simulink model "Quadcopter_Sim"  (R2020b)
settings: Solver=VariableStepAuto  StartTime=0.0  StopTime=32  RelTol=1e-3
values from neighbouring files (symbols this model uses):
  b = 1.14*10^-7    (= 1.14e-07)    [Quadcopter_Code.m]
  g = 9.81    [Quadcopter_Code.m]
  Ix = 4.856 * 10^-3    (= 0.004856)    [Quadcopter_Code.m]
  Iy = 4.856 * 10^-3    (= 0.004856)    [Quadcopter_Code.m]
  Iz = 8.801*10^-3    (= 0.008801)    [Quadcopter_Code.m]
  k = 2.98*10^-6    (= 2.98e-06)    [Quadcopter_Code.m]
  l = 0.225    [Quadcopter_Code.m]
  m = 0.468    [Quadcopter_Code.m]
libraries: pid_lib x2
settings Model: Creator=ethan  LastModifiedBy=ethan
settings OptimizationCC: BlockReduction=off  DefaultParameterBehavior=Inlined  BufferReuse=off

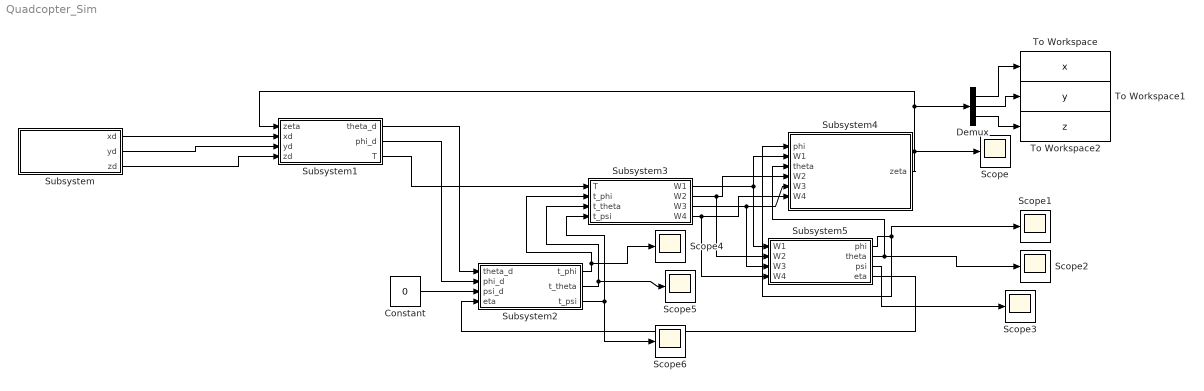
== system Quadcopter_Sim ==
  Constant : Constant  Value=0
  Demux : Demux  Outputs=3
  Scope{,1..6} (7 alike) : Scope
  Subsystem : Subsystem
  Subsystem1 : Subsystem
  Subsystem2 : Subsystem
  Subsystem3 : Subsystem
  Subsystem4 : Subsystem
  Subsystem5 : Subsystem
  To Workspace : ToWorkspace  VariableName=x  SaveFormat=Timeseries  SampleTime=-1
  To Workspace1 : ToWorkspace  VariableName=y  SaveFormat=Timeseries  SampleTime=-1
  To Workspace2 : ToWorkspace  VariableName=z  SaveFormat=Timeseries  SampleTime=-1
  wires:
  Subsystem/1(xd) -> Subsystem1/2(xd)
  Subsystem/2(yd) -> Subsystem1/3(yd)
  Subsystem/3(zd) -> Subsystem1/4(zd)
  Constant/1 -> Subsystem2/3(psi_d)
  Subsystem1/2(phi_d) -> Subsystem2/2(phi_d)
  Subsystem1/1(theta_d) -> Subsystem2/1(theta_d)
  Subsystem1/3(T) -> Subsystem3/1(T)
  Subsystem3/1(W1) -> Subsystem5/1(W1), Subsystem4/2(W1)
  Subsystem5/1(phi) -> Scope1/1, Subsystem4/1(phi)
  Subsystem4/1(zeta) -> Subsystem1/1(zeta), Demux/1, Scope/1
  Subsystem5/2(theta) -> Scope2/1, Subsystem4/3(theta)
  Subsystem5/3(psi) -> Scope3/1
  Subsystem5/4(eta) -> Subsystem2/4(eta)
  Subsystem2/1(t_phi) -> Scope4/1, Subsystem3/2(t_phi)
  Subsystem2/2(t_theta) -> Scope5/1, Subsystem3/3(t_theta)
  Subsystem2/3(t_psi) -> Subsystem3/4(t_psi), Scope6/1
  Subsystem3/2(W2) -> Subsystem5/2(W2), Subsystem4/4(W2)
  Subsystem3/3(W3) -> Subsystem4/5(W3), Subsystem5/3(W3)
  Subsystem3/4(W4) -> Subsystem5/4(W4), Subsystem4/6(W4)
  Demux/1 -> To Workspace/1
  Demux/2 -> To Workspace1/1
  Demux/3 -> To Workspace2/1

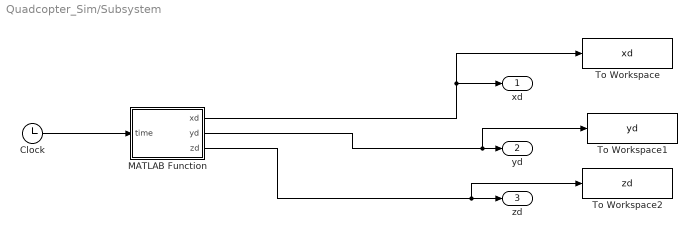
== system Quadcopter_Sim/Subsystem ==
  Clock : Clock
  MATLAB Function : MATLAB Function  TreatAsAtomicUnit=on
  To Workspace : ToWorkspace  VariableName=xd  SaveFormat=Timeseries  SampleTime=-1
  To Workspace1 : ToWorkspace  VariableName=yd  SaveFormat=Timeseries  SampleTime=-1
  To Workspace2 : ToWorkspace  VariableName=zd  SaveFormat=Timeseries  SampleTime=-1
  xd : Outport
  yd : Outport  Port=2
  zd : Outport  Port=3
  wires:
  MATLAB Function/1(xd) -> To Workspace/1, xd/1
  MATLAB Function/2(yd) -> To Workspace1/1, yd/1
  MATLAB Function/3(zd) -> To Workspace2/1, zd/1
  Clock/1 -> MATLAB Function/1(time)

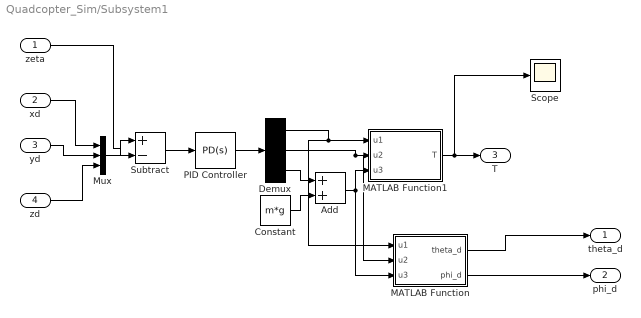
== system Quadcopter_Sim/Subsystem1 ==
  zeta : Inport
  xd : Inport  Port=2
  yd : Inport  Port=3
  zd : Inport  Port=4
  Add : Sum
  Constant : Constant  Value=m*g
  Demux : Demux  Outputs=3
  MATLAB Function : MATLAB Function  TreatAsAtomicUnit=on
  MATLAB Function1 : MATLAB Function  TreatAsAtomicUnit=on
  Mux : Mux  Inputs=3
  PID Controller : pid_lib/PID Controller  Controller=PD  Form=Parallel  TimeDomain=Continuous-time  UseExternalTs=off  SampleTime=-1  IntegratorMethod=Forward Euler  FilterMethod=Forward Euler  ControllerParametersSource=internal  P=4  I=0  D=2  UseFilter=on  N=100  TunerSelectOption=Transfer Function Based (PID Tuner App)  InitialConditionSource=internal  InitialConditionForIntegrator=0  InitialConditionForFilter=0  DifferentiatorICPrevScaledInput=0  ExternalReset=none  TrackingMode=off  Kt=1  LimitOutput=off  SatLimitsSource=internal  UpperSaturationLimit=inf  LowerSaturationLimit=-inf  LinearizeAsGain=on  AntiWindupMode=none  Kb=1  POutMin=[]  POutMax=[]  IOutMin=[]  IOutMax=[]  DOutMin=[]  DOutMax=[]  NOutMin=[]  NOutMax=[]  SumOutMin=[]  SumOutMax=[]  SaturationOutMin=[]  SaturationOutMax=[]  PParamMin=[]  PParamMax=[]  IParamMin=[]  IParamMax=[]  DParamMin=[]  DParamMax=[]  NParamMin=[]  NParamMax=[]  KbParamMin=[]  KbParamMax=[]  KtParamMin=[]  KtParamMax=[]  KbOutMin=[]  KbOutMax=[]  KtOutMin=[]  KtOutMax=[]  IntegratorOutMin=[]  IntegratorOutMax=[]  FilterOutMin=[]  FilterOutMax=[]  SumI1OutMin=[]  SumI1OutMax=[]  SumI2OutMin=[]  SumI2OutMax=[]  SumI3OutMin=[]  SumI3OutMax=[]  SumI4OutMin=[]  SumI4OutMax=[]  SumDOutMin=[]  SumDOutMax=[]  DifferentiatorOutMin=[]  DifferentiatorOutMax=[]  FilterDiffOutCoefMin=[]  FilterDiffOutCoefMax=[]  ReciprocalOutMin=[]  ReciprocalOutMax=[]  SumDenOutMin=[]  SumDenOutMax=[]  SumNumOutMin=[]  SumNumOutMax=[]  DivideOutMin=[]  DivideOutMax=[]  UdiffTsProdOutMin=[]  UdiffTsProdOutMax=[]  NTsProdOutMin=[]  NTsProdOutMax=[]  UintegralTsProdOutMin=[]  UintegralTsProdOutMax=[]  UngainTsProdOutMin=[]  UngainTsProdOutMax=[]  IntegratorContinuousStateAttributes=''  IntegratorStateMustResolveToSignalObject=off  IntegratorRTWStateStorageClass=Auto  FilterContinuousStateAttributes=''  FilterStateMustResolveToSignalObject=off  FilterRTWStateStorageClass=Auto  ParallelPVariant=InternalParameters  IdealPVariant=Disabled  IVariant=Disabled  DVariant=InternalParameters  IntegratorVariant=Disabled  SatVariant=Disabled  AWVariant=Disabled  PCopyVariant=Disabled  TRVariant=Disabled  FdbkBlocksVariant=Forward  IdealPFdbkVariant=Disabled  SatFdbkVariant=Disabled  DerivativeFilterVariant=ContFilter  NVariant=InternalParameters  NCopyVariant=Disabled  FilterICVariant=InternalICsFilter  IntegratorICVariant=Disabled  ExternalResetVariant=Disabled  TRSumVariant=Passthrough  SumFdbkVariant=Disabled  SumVariant=Sum_PD  TsampFilterVariant=InternalTs  TsampNgainVariant=Passthrough  TsampIntegralVariant=Disabled_SignalSpec  ExternalSaturationOutDataTypeStr=Inherit: Same as second input
  Scope : Scope
  Subtract : Sum  Inputs=+-
  theta_d : Outport
  phi_d : Outport  Port=2
  T : Outport  Port=3
  wires:
  xd/1 -> Mux/1
  yd/1 -> Mux/2
  zd/1 -> Mux/3
  zeta/1 -> Subtract/2
  Mux/1 -> Subtract/1
  Subtract/1 -> PID Controller/1
  PID Controller/1 -> Demux/1
  MATLAB Function/1(theta_d) -> theta_d/1
  MATLAB Function/2(phi_d) -> phi_d/1
  Demux/3 -> Add/1
  Add/1 -> MATLAB Function1/3(u3), MATLAB Function/3(u3)
  Demux/2 -> MATLAB Function/2(u2), MATLAB Function1/2(u2)
  Demux/1 -> MATLAB Function1/1(u1), MATLAB Function/1(u1)
  MATLAB Function1/1(T) -> Scope/1, T/1
  Constant/1 -> Add/2

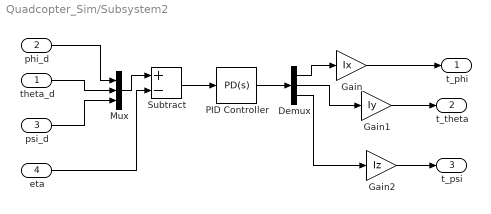
== system Quadcopter_Sim/Subsystem2 ==
  theta_d : Inport
  phi_d : Inport  Port=2
  psi_d : Inport  Port=3
  eta : Inport  Port=4
  Demux : Demux  Outputs=3
  Gain : Gain  Gain=Ix
  Gain1 : Gain  Gain=Iy
  Gain2 : Gain  Gain=Iz
  Mux : Mux  Inputs=3
  PID Controller : pid_lib/PID Controller  Controller=PD  Form=Parallel  TimeDomain=Continuous-time  UseExternalTs=off  SampleTime=-1  IntegratorMethod=Forward Euler  FilterMethod=Forward Euler  ControllerParametersSource=internal  P=1  I=0  D=3  UseFilter=on  N=100  TunerSelectOption=Transfer Function Based (PID Tuner App)  InitialConditionSource=internal  InitialConditionForIntegrator=0  InitialConditionForFilter=0  DifferentiatorICPrevScaledInput=0  ExternalReset=none  TrackingMode=off  Kt=1  LimitOutput=off  SatLimitsSource=internal  UpperSaturationLimit=inf  LowerSaturationLimit=-inf  LinearizeAsGain=on  AntiWindupMode=none  Kb=1  POutMin=[]  POutMax=[]  IOutMin=[]  IOutMax=[]  DOutMin=[]  DOutMax=[]  NOutMin=[]  NOutMax=[]  SumOutMin=[]  SumOutMax=[]  SaturationOutMin=[]  SaturationOutMax=[]  PParamMin=[]  PParamMax=[]  IParamMin=[]  IParamMax=[]  DParamMin=[]  DParamMax=[]  NParamMin=[]  NParamMax=[]  KbParamMin=[]  KbParamMax=[]  KtParamMin=[]  KtParamMax=[]  KbOutMin=[]  KbOutMax=[]  KtOutMin=[]  KtOutMax=[]  IntegratorOutMin=[]  IntegratorOutMax=[]  FilterOutMin=[]  FilterOutMax=[]  SumI1OutMin=[]  SumI1OutMax=[]  SumI2OutMin=[]  SumI2OutMax=[]  SumI3OutMin=[]  SumI3OutMax=[]  SumI4OutMin=[]  SumI4OutMax=[]  SumDOutMin=[]  SumDOutMax=[]  DifferentiatorOutMin=[]  DifferentiatorOutMax=[]  FilterDiffOutCoefMin=[]  FilterDiffOutCoefMax=[]  ReciprocalOutMin=[]  ReciprocalOutMax=[]  SumDenOutMin=[]  SumDenOutMax=[]  SumNumOutMin=[]  SumNumOutMax=[]  DivideOutMin=[]  DivideOutMax=[]  UdiffTsProdOutMin=[]  UdiffTsProdOutMax=[]  NTsProdOutMin=[]  NTsProdOutMax=[]  UintegralTsProdOutMin=[]  UintegralTsProdOutMax=[]  UngainTsProdOutMin=[]  UngainTsProdOutMax=[]  IntegratorContinuousStateAttributes=''  IntegratorStateMustResolveToSignalObject=off  IntegratorRTWStateStorageClass=Auto  FilterContinuousStateAttributes=''  FilterStateMustResolveToSignalObject=off  FilterRTWStateStorageClass=Auto  ParallelPVariant=InternalParameters  IdealPVariant=Disabled  IVariant=Disabled  DVariant=InternalParameters  IntegratorVariant=Disabled  SatVariant=Disabled  AWVariant=Disabled  PCopyVariant=Disabled  TRVariant=Disabled  FdbkBlocksVariant=Forward  IdealPFdbkVariant=Disabled  SatFdbkVariant=Disabled  DerivativeFilterVariant=ContFilter  NVariant=InternalParameters  NCopyVariant=Disabled  FilterICVariant=InternalICsFilter  IntegratorICVariant=Disabled  ExternalResetVariant=Disabled  TRSumVariant=Passthrough  SumFdbkVariant=Disabled  SumVariant=Sum_PD  TsampFilterVariant=InternalTs  TsampNgainVariant=Passthrough  TsampIntegralVariant=Disabled_SignalSpec  ExternalSaturationOutDataTypeStr=Inherit: Same as second input
  Subtract : Sum  Inputs=+-
  t_phi : Outport
  t_theta : Outport  Port=2
  t_psi : Outport  Port=3
  wires:
  phi_d/1 -> Mux/1
  theta_d/1 -> Mux/2
  psi_d/1 -> Mux/3
  Mux/1 -> Subtract/1
  eta/1 -> Subtract/2
  Subtract/1 -> PID Controller/1
  PID Controller/1 -> Demux/1
  Demux/1 -> Gain/1
  Gain/1 -> t_phi/1
  Gain1/1 -> t_theta/1
  Demux/2 -> Gain1/1
  Gain2/1 -> t_psi/1
  Demux/3 -> Gain2/1

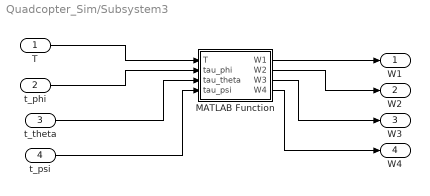
== system Quadcopter_Sim/Subsystem3 ==
  T : Inport
  t_phi : Inport  Port=2
  t_theta : Inport  Port=3
  t_psi : Inport  Port=4
  MATLAB Function : MATLAB Function  TreatAsAtomicUnit=on
  W1 : Outport
  W2 : Outport  Port=2
  W3 : Outport  Port=3
  W4 : Outport  Port=4
  wires:
  MATLAB Function/1(W1) -> W1/1
  T/1 -> MATLAB Function/1(T)
  t_phi/1 -> MATLAB Function/2(tau_phi)
  t_theta/1 -> MATLAB Function/3(tau_theta)
  t_psi/1 -> MATLAB Function/4(tau_psi)
  MATLAB Function/2(W2) -> W2/1
  MATLAB Function/3(W3) -> W3/1
  MATLAB Function/4(W4) -> W4/1

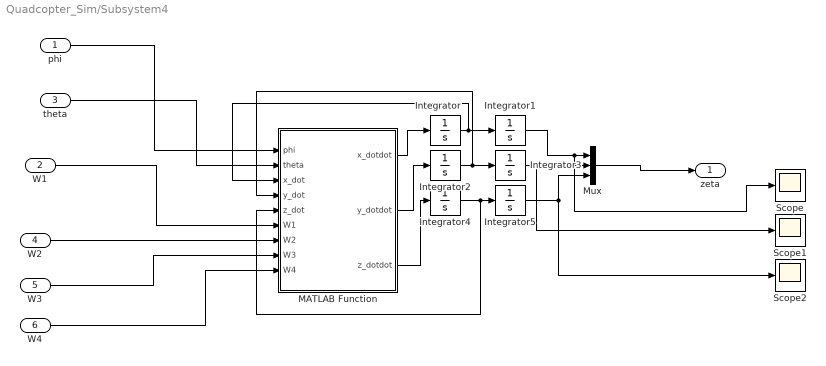
== system Quadcopter_Sim/Subsystem4 ==
  phi : Inport
  W1 : Inport  Port=2
  theta : Inport  Port=3
  W2 : Inport  Port=4
  W3 : Inport  Port=5
  W4 : Inport  Port=6
  Integrator{,1..4} (5 alike) : Integrator
  Integrator5 : Integrator  InitialCondition=3
  MATLAB Function : MATLAB Function  TreatAsAtomicUnit=on
  Mux : Mux  Inputs=3
  Scope : Scope
  Scope1 : Scope
  Scope2 : Scope
  zeta : Outport
  wires:
  W1/1 -> MATLAB Function/6(W1)
  MATLAB Function/1(x_dotdot) -> Integrator/1
  Integrator/1 -> Integrator1/1, MATLAB Function/3(x_dot)
  theta/1 -> MATLAB Function/2(theta)
  phi/1 -> MATLAB Function/1(phi)
  Mux/1 -> zeta/1
  Integrator1/1 -> Scope/1, Mux/1
  MATLAB Function/2(y_dotdot) -> Integrator2/1
  Integrator2/1 -> MATLAB Function/4(y_dot), Integrator3/1
  Integrator3/1 -> Scope1/1, Mux/2
  MATLAB Function/3(z_dotdot) -> Integrator4/1
  Integrator4/1 -> MATLAB Function/5(z_dot), Integrator5/1
  Integrator5/1 -> Scope2/1, Mux/3
  W2/1 -> MATLAB Function/7(W2)
  W3/1 -> MATLAB Function/8(W3)
  W4/1 -> MATLAB Function/9(W4)

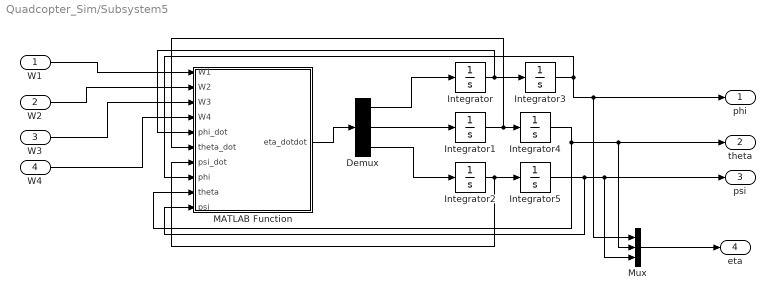
== system Quadcopter_Sim/Subsystem5 ==
  W1 : Inport
  W2 : Inport  Port=2
  W3 : Inport  Port=3
  W4 : Inport  Port=4
  Demux : Demux  Outputs=3
  Integrator{,1..5} (6 alike) : Integrator
  MATLAB Function : MATLAB Function  TreatAsAtomicUnit=on
  Mux : Mux  Inputs=3
  phi : Outport
  theta : Outport  Port=2
  psi : Outport  Port=3
  eta : Outport  Port=4
  wires:
  W1/1 -> MATLAB Function/1(W1)
  MATLAB Function/1(eta_dotdot) -> Demux/1
  Demux/1 -> Integrator/1
  Demux/2 -> Integrator1/1
  Demux/3 -> Integrator2/1
  Integrator/1 -> Integrator3/1, MATLAB Function/5(phi_dot)
  Integrator1/1 -> MATLAB Function/6(theta_dot), Integrator4/1
  Integrator2/1 -> Integrator5/1, MATLAB Function/7(psi_dot)
  Integrator3/1 -> Mux/1, phi/1, MATLAB Function/8(phi)
  Integrator4/1 -> Mux/2, theta/1, MATLAB Function/9(theta)
  Integrator5/1 -> Mux/3, psi/1, MATLAB Function/10(psi)
  Mux/1 -> eta/1
  W2/1 -> MATLAB Function/2(W2)
  W3/1 -> MATLAB Function/3(W3)
  W4/1 -> MATLAB Function/4(W4)

== matlab function Quadcopter_Sim/Subsystem1/MATLAB Function1 ==
  data: u1 input; T output; u2 input; u3 input
function T = fcn(u1, u2, u3)
T = sqrt(u1^2 + u2^2 + u3^2);
end

== matlab function Quadcopter_Sim/Subsystem1/MATLAB Function ==
  data: u1 input; theta_d output; phi_d output; u2 input; u3 input
function [theta_d, phi_d] = fcn(u1,u2,u3)
theta_d = atan(u1/(u3));
phi_d = atan((-u2*cos(theta_d))/(u3));
end

== matlab function Quadcopter_Sim/Subsystem3/MATLAB Function ==
  data: T input; W1 output; tau_phi input; tau_theta input; tau_psi input; W2 output; W3 output; W4 output
function [W1,W2,W3,W4] = fcn(T, tau_phi, tau_theta, tau_psi)
k = 2.98*10^-6;
b = 1.14*10^-7;
l = 0.225;

W1 = T/(4*k) - tau_theta/(2*k*l) - tau_psi/(4*b);
W2 = T/(4*k) - tau_phi/(2*k*l) + tau_psi/(4*b);
W3 = T/(4*k) + tau_theta/(2*k*l) - tau_psi/(4*b);
W4 = T/(4*k) + tau_phi/(2*k*l) + tau_psi/(4*b);
end

== matlab function Quadcopter_Sim/Subsystem5/MATLAB Function ==
  data: W1 input; W2 input; W3 input; W4 input; eta_dotdot output; phi_dot input; theta_dot input; psi_dot input; phi input; theta input; psi input; l parameter; k parameter; b parameter
function eta_dotdot  = fcn(W1, W2, W3, W4, phi_dot, theta_dot, psi_dot, phi, theta, psi, l, k, b)
k = 2.980000000000000e-06;
l = 0.225;
b = 1.14 * 10^-7;




Ix = 4.856*10^-3;
Iy = 4.856*10^-3;
Iz = 8.801*10^-3;

tau_phi = l * k * (-W2 + W4);
tau_theta = l* k* (-W1 + W3);
tau_psi = b * (-W1 +W2 -W3 + W4);

J = zeros(3,3);
C = zeros(3,3);

J(1,1) = Ix;
J(1,3) = -Ix * sin(theta);
J(2,2) = Iy*(cos(phi))^2+Iz*(sin(phi))^2;
J(2,3) = (Iy-Iz)*cos(phi)*sin(phi)*cos(theta);
J(3,1) = -Ix*sin(theta);
J(3,2) = (Iy-Iz)*cos(phi)*sin(phi)*cos(theta);
J(3,3) = Ix*(sin(theta))^2+Iy*(sin(phi))^2*(cos(theta))^2+Iz*cos(phi)^2*cos(theta)^2;

C(1,2) = (Iy-Iz)*(theta_dot*cos(phi)*sin(phi)+psi_dot*(sin(phi))^2*cos(theta))+...
    (Iz-Iy)*psi_dot*(cos(phi))^2*cos(theta)-Ix*psi_dot*cos(theta);
C(1,3) = (Iz-Iy)*psi_dot*cos(phi)*sin(phi)*(cos(theta))^2;
C(2,1) = (Iz-Iy)*(theta_dot*cos(phi)*sin(phi)+psi_dot*sin(phi)*cos(theta))+...
    (Iy-Iz)*psi_dot*(cos(phi))^2*cos(theta)+Ix*psi_dot*cos(theta);
C(2,2) = (Iz-Iy)*phi_dot*cos(phi)*sin(phi);
C(2,3) = -Iz*psi_dot*sin(theta)*cos(theta)+Iy*psi_dot*(sin(phi)^2*sin(theta)*cos(theta))+...
    Iz*psi_dot*(cos(phi))^2*sin(theta)*cos(theta);
C(3,1) = (Iy-Iz)*psi_dot*(cos(theta))^2*sin(phi)*cos(phi)-Ix*theta_dot*cos(theta);
C(3,2) = (Iz-Iy)*(theta_dot*cos(phi)*sin(phi)*sin(theta)+phi_dot*(sin(phi))^2*cos(theta))+...
    (Iy-Iz)*phi_dot*(cos(phi))^2*cos(theta)+Ix*psi_dot*sin(theta)*cos(theta)-...
    Iy*psi_dot*(sin(phi))^2*sin(theta)*cos(theta)-Iz*psi_dot*(cos(phi))^2*sin(theta)*cos(theta);
C(3,3) = (Iy-Iz)*phi_dot*cos(phi)*sin(phi)*(cos(theta))^2-Iy*theta_dot*(sin(phi))^2*cos(theta)*sin(theta)-...
    Iz*theta_dot*(cos(phi))^2*cos(theta)*sin(theta)+Ix*theta_dot*cos(theta)*sin(theta);

B = [tau_phi tau_theta tau_psi]';
N = [phi_dot theta_dot psi_dot]';

eta_dotdot = inv(J) * (B - C*N);
end

== matlab function Quadcopter_Sim/Subsystem4/MATLAB Function ==
  data: phi input; theta input; x_dotdot output; x_dot input; y_dot input; z_dot input; W1 input; y_dotdot output; z_dotdot output; W2 input; W3 input; W4 input
function [x_dotdot, y_dotdot, z_dotdot] = fcn(phi, theta, x_dot, y_dot, z_dot, W1, W2, W3, W4)
m = 0.468;
g = 9.81;
Ax = 0.25;
Ay = 0.25;
Az = 0.25;
k = 2.98*10^-6;

T = k*(W1+W2+W3+W4);

x_dotdot = T/m*cos(phi)*sin(theta) - Ax/m * x_dot;
y_dotdot = T/m * -sin(phi) - Ay/m * y_dot;
z_dotdot = T/m*cos(phi)*cos(theta) - g - Az/m * z_dot;
end

== matlab function Quadcopter_Sim/Subsystem/MATLAB Function ==
  data: time input; xd output; yd output; zd output
function [xd, yd, zd] = fcn(time)
if time <= 10
xd = time;
yd = 0;
zd = (time * 0.5) + 3;
elseif time <= 18 
xd = cos(time - 10) + 9;
yd = sin(time - 10);
zd = 8 + (time-10)*0.5;
else
xd = (cos(8)) + 9 - (time - 18);
yd = (sin(8));
zd = 12 - ((time-18)*9/14);
end
